simulink model "uav_kinematics"  (R2021a)
settings: Solver=VariableStepAuto  StartTime=0.0  StopTime=Inf  RelTol=1e-3
undefined symbols (not defined in the file or in its folder): drawAircraft
libraries: simulink x6
settings Model: Creator=Duncan Gichuru  LastModifiedBy=dunca

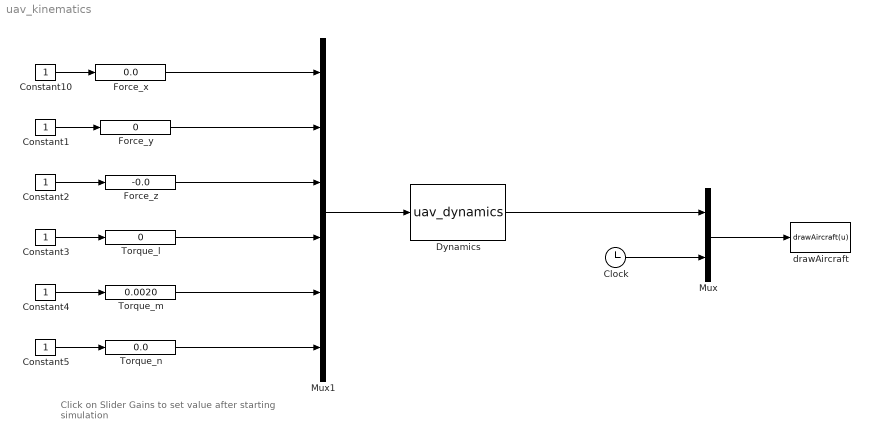
== system uav_kinematics ==
  note: Click on Slider Gains to set value
      | after starting simulation
  Clock : Clock
  Constant{1..5,10} (6 alike) : Constant
  Dynamics : S-Function  FunctionName=uav_dynamics  Parameters=UAV  SFunctionDeploymentMode=off  EnableBusSupport=off
  Force_x : simulink/Math Operations/Slider Gain  gain=0.0  low=-1  high=1
  Force_y : simulink/Math Operations/Slider Gain  gain=0  low=-1  high=1
  Force_z : simulink/Math Operations/Slider Gain  gain=-0.0  low=-1  high=1
  Mux : Mux  Inputs=2
  Mux1 : Mux  Inputs=6
  Torque_l : simulink/Math Operations/Slider Gain  gain=0  low=-0.1  high=0.1
  Torque_m : simulink/Math Operations/Slider Gain  gain=0.0020  low=-0.1  high=0.1
  "Torque_n " : simulink/Math Operations/Slider Gain  gain=0.0  low=-0.1  high=0.1
  drawAircraft : MATLABFcn  MATLABFcn=drawAircraft(u)  OutputDimensions=0  SampleTime=0.1
  wires:
  "Torque_n "/1 -> Mux1/6
  Constant3/1 -> Torque_l/1
  Force_x/1 -> Mux1/1
  Mux1/1 -> Dynamics/1
  Torque_l/1 -> Mux1/4
  Constant4/1 -> Torque_m/1
  Constant2/1 -> Force_z/1
  Torque_m/1 -> Mux1/5
  Force_y/1 -> Mux1/2
  Force_z/1 -> Mux1/3
  Constant1/1 -> Force_y/1
  Constant5/1 -> "Torque_n "/1
  Constant10/1 -> Force_x/1
  Mux/1 -> drawAircraft/1
  Clock/1 -> Mux/2
  Dynamics/1 -> Mux/1
